simulink model "Yaw_LQIDG"  (R2020a)
settings: Solver=ode3  StartTime=0.0  StopTime=10  FixedStep=0.02  RelTol=1e-3
InitFcn:
  | OpenLoop_LQDG_riccati_solver
values from neighbouring files (symbols this model uses):
  LQIDG_openloop_gain = (R1_inv * B' * p1)    [OpenLoop_LQDG_riccati_solver.m]
undefined symbols (not defined in the file or in its folder): A3, B3, C2, C3, magnitude
libraries: simulink x1
settings Model: Creator=Ali  LastModifiedBy=Ali

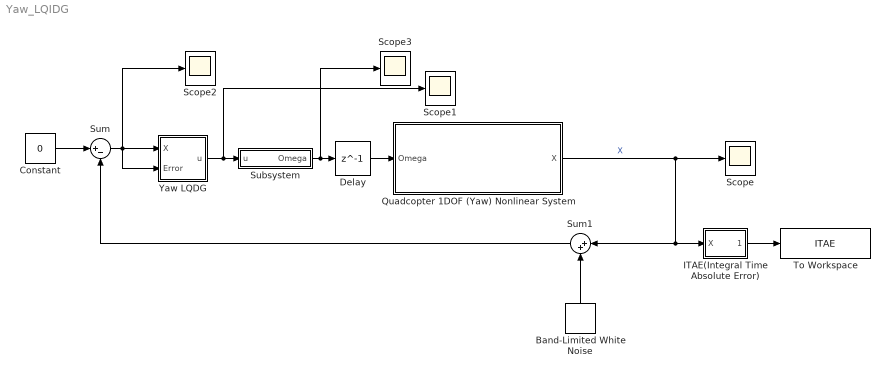
== system Yaw_LQIDG ==
  Band-Limited White Noise : simulink/Sources/Band-Limited White Noise  Cov=[0.0001]  Ts=0.02  seed=[23341]
  Constant : Constant  Value=0
  Delay : Delay  DelayLength=1
  ITAE(Integral Time Absolute Error) : Subsystem
  Quadcopter 1DOF (Yaw) Nonlinear System : Subsystem  TreatAsAtomicUnit=on
      mask Display: image('quad1.png'); % Use "Edit Image" on toolstrip to change.
  Scope{,1..3} (4 alike) : Scope
  Subsystem : Subsystem
  Sum : Sum  Inputs=|+-
  Sum1 : Sum  Inputs=|++
  To Workspace : ToWorkspace  VariableName=ITAE  SaveFormat=Timeseries  SampleTime=-1
  Yaw LQDG : Subsystem
  wires:
  Quadcopter 1DOF (Yaw) Nonlinear System/1(X) -> Sum1/1, ITAE(Integral Time Absolute Error)/1(X), Scope/1  "X"
  Constant/1 -> Sum/1
  ITAE(Integral Time Absolute Error)/1(ITAE) -> To Workspace/1
  Band-Limited White Noise/1 -> Sum1/2
  Yaw LQDG/1(u) -> Scope1/1, Subsystem/1(u)
  Sum/1 -> Scope2/1, Yaw LQDG/2(Error), Yaw LQDG/1(X)
  Sum1/1 -> Sum/2
  Subsystem/1(Omega) -> Scope3/1, Delay/1
  Delay/1 -> Quadcopter 1DOF (Yaw) Nonlinear System/1(Omega)

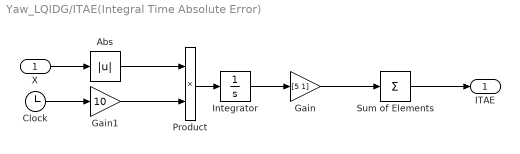
== system Yaw_LQIDG/ITAE(Integral Time Absolute Error) ==
  X : Inport
  Abs : Abs
  Clock : Clock
  Gain : Gain  Gain=[5 1]
  Gain1 : Gain  Gain=10
  Integrator : Integrator
  Product : Product
  Sum of Elements : Sum  Inputs=+
  ITAE : Outport
  wires:
  Product/1 -> Integrator/1
  Integrator/1 -> Gain/1
  Clock/1 -> Gain1/1
  Sum of Elements/1 -> ITAE/1
  Abs/1 -> Product/1
  X/1 -> Abs/1
  Gain/1 -> Sum of Elements/1
  Gain1/1 -> Product/2

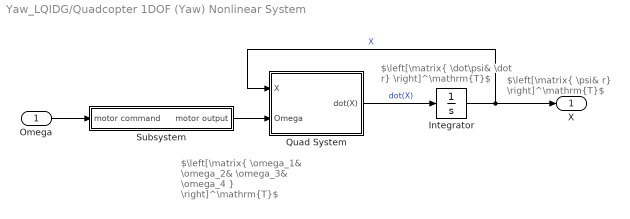
== system Yaw_LQIDG/Quadcopter 1DOF (Yaw) Nonlinear System ==
  note: $\left[\matrix{ \dot\psi& \dot r} \right]^\mathrm{T}$
  note: $\left[\matrix{ \omega_1& \omega_2& \omega_3& \omega_4 } \right]^\mathrm{T}$
  note: $\left[\matrix{ \psi& r} \right]^\mathrm{T}$
  Omega : Inport
  Integrator : Integrator  InitialCondition=[1.5, 0]
  Quad System : Subsystem
  Subsystem : Subsystem
  X : Outport
  wires:
  Integrator/1 -> Quad System/1(X), X/1  "X"
  Quad System/1(dot(X)) -> Integrator/1  "dot(X)"
  Omega/1 -> Subsystem/1(motor command)
  Subsystem/1(motor output) -> Quad System/2(Omega)

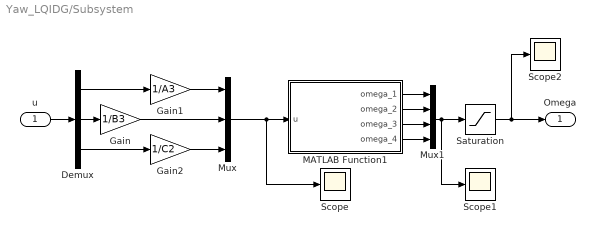
== system Yaw_LQIDG/Subsystem ==
  u : Inport
  Demux : Demux  Outputs=3
  Gain : Gain  Gain=1/B3
  Gain1 : Gain  Gain=1/A3
  Gain2 : Gain  Gain=1/C2
  MATLAB Function1 : MATLAB Function  TreatAsAtomicUnit=on
  Mux : Mux  Inputs=3
  Mux1 : Mux
  Saturation : Saturate  UpperLimit=6000/60*2*pi  LowerLimit=1300/60*2*pi
  Scope : Scope
  Scope1 : Scope
  Scope2 : Scope
  Omega : Outport
  wires:
  MATLAB Function1/1(omega_1) -> Mux1/1
  MATLAB Function1/2(omega_2) -> Mux1/2
  MATLAB Function1/4(omega_4) -> Mux1/4
  MATLAB Function1/3(omega_3) -> Mux1/3
  Mux1/1 -> Scope1/1, Saturation/1
  Mux/1 -> Scope/1, MATLAB Function1/1(u)
  Gain/1 -> Mux/2
  Gain1/1 -> Mux/1
  u/1 -> Demux/1
  Demux/2 -> Gain/1
  Demux/1 -> Gain1/1
  Demux/3 -> Gain2/1
  Gain2/1 -> Mux/3
  Saturation/1 -> Scope2/1, Omega/1

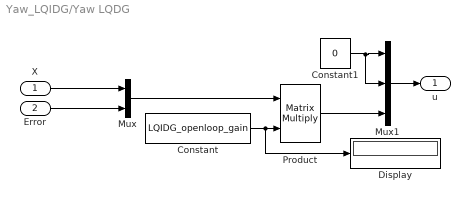
== system Yaw_LQIDG/Yaw LQDG ==
  X : Inport
  Error : Inport  Port=2
  Constant : Constant  Value=LQIDG_openloop_gain
  Constant1 : Constant  Value=0
  Display : Display
  Mux : Mux  Inputs=2
  Mux1 : Mux  Inputs=3
  Product : Product  Multiplication=Matrix(*)
  u : Outport
  wires:
  Constant/1 -> Display/1, Product/2
  X/1 -> Mux/1
  Error/1 -> Mux/2
  Mux/1 -> Product/1
  Product/1 -> Mux1/3
  Mux1/1 -> u/1
  Constant1/1 -> Mux1/1, Mux1/2

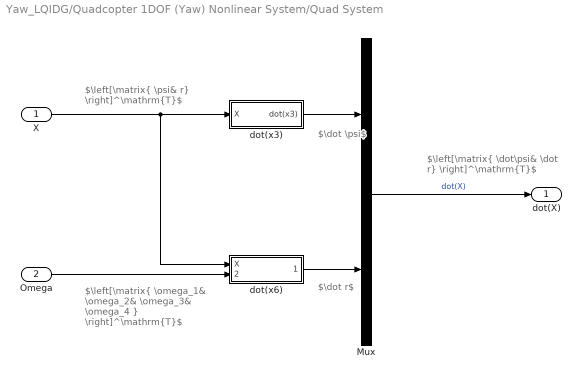
== system Yaw_LQIDG/Quadcopter 1DOF (Yaw) Nonlinear System/Quad System ==
  note: $\left[\matrix{ \omega_1& \omega_2& \omega_3& \omega_4 } \right]^\mathrm{T}$
  note: $\left[\matrix{ \dot\psi& \dot r} \right]^\mathrm{T}$
  note: $\dot \psi$
  note: $\dot r$
  note: $\left[\matrix{ \psi& r} \right]^\mathrm{T}$
  X : Inport
  Omega : Inport  Port=2
  Mux : Mux  Inputs=2
  dot(x3) : Subsystem
  dot(x6) : Subsystem
  dot(X) : Outport
  wires:
  Mux/1 -> dot(X)/1  "dot(X)"
  X/1 -> dot(x6)/1(X), dot(x3)/1(X)
  Omega/1 -> dot(x6)/2(Omega)
  dot(x3)/1(dot(x3)) -> Mux/1
  dot(x6)/1(dot(x6)) -> Mux/2

== system Yaw_LQIDG/Quadcopter 1DOF (Yaw) Nonlinear System/Subsystem ==
  motor command : Inport
  For Each Subsystem : Subsystem  TreatAsAtomicUnit=on
  motor output : Outport
  wires:
  motor command/1 -> For Each Subsystem/1(Omega_c)
  For Each Subsystem/1(Omega_m) -> motor output/1

== system Yaw_LQIDG/Quadcopter 1DOF (Yaw) Nonlinear System/Quad System/dot(x3) ==
  X : Inport
  Subsystem : Subsystem
  dot(x3) : Outport
  wires:
  X/1 -> Subsystem/1(X)  "X"
  Subsystem/1(x6cos(x1)) -> dot(x3)/1

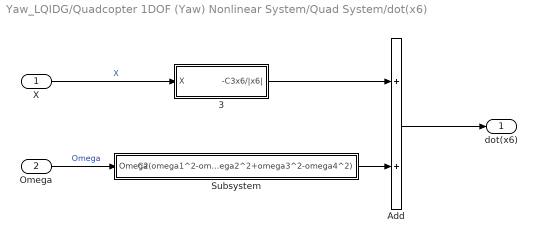
== system Yaw_LQIDG/Quadcopter 1DOF (Yaw) Nonlinear System/Quad System/dot(x6) ==
  X : Inport
  Omega : Inport  Port=2
  3 : Subsystem
  Add : Sum
  Subsystem : Subsystem
  dot(x6) : Outport
  wires:
  Omega/1 -> Subsystem/1(Omega)  "Omega"
  Add/1 -> dot(x6)/1
  3/1("-C3x6/|x6| ") -> Add/1
  X/1 -> 3/1(X)  "X"
  Subsystem/1(C2(omega1^2-omega2^2+omega3^2-omega4^2)) -> Add/2

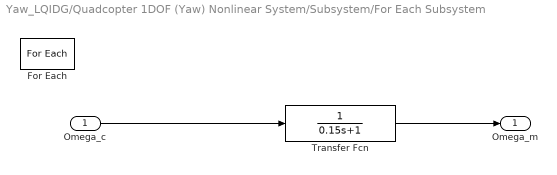
== system Yaw_LQIDG/Quadcopter 1DOF (Yaw) Nonlinear System/Subsystem/For Each Subsystem ==
  Omega_c : Inport  Partition=on  PartitionDimension=1  PartitionWidth=1  PartitionOffset=0
  For Each : ForEach  DisableCoverage=on
  Transfer Fcn : TransferFcn  Denominator=[0.15 1]
  Omega_m : Outport  ConcatenationDimension=1
  wires:
  Omega_c/1 -> Transfer Fcn/1
  Transfer Fcn/1 -> Omega_m/1

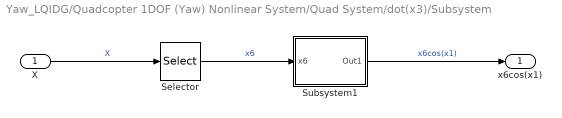
== system Yaw_LQIDG/Quadcopter 1DOF (Yaw) Nonlinear System/Quad System/dot(x3)/Subsystem ==
  X : Inport
  Selector : Selector  InputPortWidth=2  IndexOptions=Index vector (dialog)  Indices=[2]  OutputSizes=1
  Subsystem1 : Subsystem
  x6cos(x1) : Outport
  wires:
  Selector/1 -> Subsystem1/1(x6)  "x6"
  Subsystem1/1(Out1) -> x6cos(x1)/1  "x6cos(x1)"
  X/1 -> Selector/1  "X"

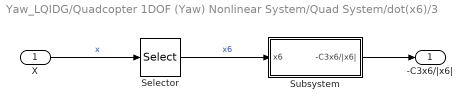
== system Yaw_LQIDG/Quadcopter 1DOF (Yaw) Nonlinear System/Quad System/dot(x6)/3 ==
  X : Inport
  Selector : Selector  InputPortWidth=2  IndexOptions=Index vector (dialog)  Indices=[2]  OutputSizes=1
  Subsystem : Subsystem
  "-C3x6/|x6| " : Outport
  wires:
  Selector/1 -> Subsystem/1(x6)  "x6"
  Subsystem/1("-C3x6/|x6| ") -> "-C3x6/|x6| "/1
  X/1 -> Selector/1  "x"

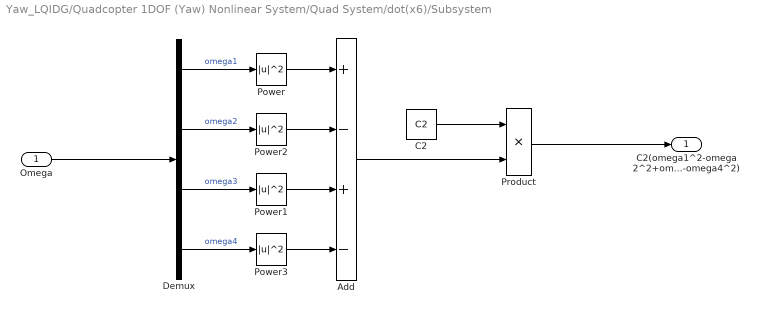
== system Yaw_LQIDG/Quadcopter 1DOF (Yaw) Nonlinear System/Quad System/dot(x6)/Subsystem ==
  Omega : Inport
  Add : Sum  Inputs=+-+-
  C2 : Constant  Value=C2
  Demux : Demux
  Power{,1..3} (4 alike) : Math  Operator=magnitude^2  SaturateOnIntegerOverflow=on
  Product : Product
  C2(omega1^2-omega2^2+omega3^2-omega4^2) : Outport
  wires:
  Omega/1 -> Demux/1
  Demux/3 -> Power1/1  "omega3"
  Demux/1 -> Power/1  "omega1"
  Demux/2 -> Power2/1  "omega2"
  Demux/4 -> Power3/1  "omega4"
  C2/1 -> Product/1
  Add/1 -> Product/2
  Product/1 -> C2(omega1^2-omega2^2+omega3^2-omega4^2)/1
  Power/1 -> Add/1
  Power2/1 -> Add/2
  Power1/1 -> Add/3
  Power3/1 -> Add/4

== system Yaw_LQIDG/Quadcopter 1DOF (Yaw) Nonlinear System/Quad System/dot(x3)/Subsystem/Subsystem1 ==
  x6 : Inport
  Out1 : Outport
  wires:
  x6/1 -> Out1/1

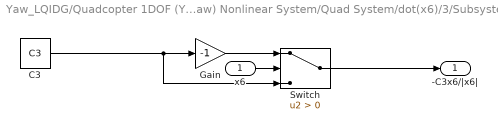
== system Yaw_LQIDG/Quadcopter 1DOF (Yaw) Nonlinear System/Quad System/dot(x6)/3/Subsystem ==
  x6 : Inport
  C3 : Constant  Value=C3
  Gain : Gain  Gain=-1
  Switch : Switch  Criteria=u2 > Threshold
  "-C3x6/|x6| " : Outport
  wires:
  Switch/1 -> "-C3x6/|x6| "/1
  C3/1 -> Switch/3, Gain/1
  x6/1 -> Switch/2
  Gain/1 -> Switch/1

== matlab function Yaw_LQIDG/Subsystem/MATLAB Function1 ==
  data: u input size=3; omega_1 output size=1; omega_2 output size=1; omega_3 output size=1; omega_4 output size=1
function [omega_1, omega_2, omega_3, omega_4] = fcn(u)
u1 = u(1);
u2 = u(2);
u3 = u(3);
% control effort
u4 = ones(1, length(u1)) * 4 * rpm2rad_sec(2000)^2;
% calculate omega
if (u4 + u3 + 2 * u2) / 4 > 0
    omega_1 = sqrt((u4 + u3 + 2 * u2) / 4);
else
    omega_1 = 0;
end
if (u4 + u3 - 2 * u2) / 4 > 0
    omega_3 = sqrt((u4 + u3 - 2 * u2) / 4);
else
    omega_3 = 0;
end
if (u4 - u3 + 2 * u1) / 4 > 0
    omega_2 = sqrt((u4 - u3 + 2 * u1) / 4);
else
    omega_2 = 0;
end
if (u4 - u3 - 2 * u1) / 4 > 0
    omega_4 = sqrt((u4 - u3 - 2 * u1) / 4);
else
    omega_4 = 0;
end
end
%% functions
% rpm to rad/sec
function rad = rpm2rad_sec(rpm)
rad = rpm / 60 * 2 * pi;
end
